simulink model "Airship_nonlinear_dynamics_simulink"  (R2024b)
settings: Solver=ode15s  StartTime=0.0  StopTime=1000  FixedStep=0.01  MaxStep=0.01  RelTol=1e-5  AbsTol=1e-8
InitFcn:
  | Init
values from neighbouring files (symbols this model uses):
  c = 0.465    [Init.m]    (also in Nonlinear_dynamics.m = 7; init_Skyship.m = 7)
  cf = 0.1395    [Init.m]    (also in Nonlinear_dynamics.m = 3; init_Skyship.m = 3)
  CL_alpha = 5.7    [Init.m]    (also in Nonlinear_dynamics.m; init_Skyship.m)
  D = 1.6    [Init.m]    (also in Nonlinear_dynamics.m = 14; init_Skyship.m = 14)
  delta = deg2rad(10)    [Nonlinear_dynamics.m]    (also in init_Skyship.m = -15)
  delta_e = 0    [Init.m]
  delta_r = 0    [Init.m]
  etaTDF = 1    [Init.m]    (also in Nonlinear_dynamics.m = 0.6; init_Skyship.m = 0.6)
  etaTP = 0.6    [Init.m]    (also in Nonlinear_dynamics.m; init_Skyship.m)
  fProp1 = 0    [Init.m]
  fProp2 = 0    [Init.m]
  fProp_max = 20    [Init.m]
  fTDF = 4000    [Nonlinear_dynamics.m]    (also in init_Skyship.m = 0)
  fTTP = 0    [Init.m]    (also in Nonlinear_dynamics.m = 2000; init_Skyship.m)
  FVN = [5, 5, 5]    [Init.m]    (also in Nonlinear_dynamics.m = 0; init_Skyship.m = 10)
  g = 9.81    [Init.m]    (also in Nonlinear_dynamics.m; init_Skyship.m)
  I33 = eye(3)    [Init.m]    (also in Nonlinear_dynamics.m; init_Skyship.m)
  Ixx = 1.7972    [Init.m]    (also in Nonlinear_dynamics.m = 200658; init_Skyship.m = 200658)
  Ixy = 0    [Init.m]    (also in Nonlinear_dynamics.m; init_Skyship.m)
  Ixz = 0    [Init.m]    (also in Nonlinear_dynamics.m; init_Skyship.m)
  Iyy = 4.9584    [Init.m]    (also in Nonlinear_dynamics.m = 850900; init_Skyship.m = 850900)
  Iyz = 0    [Init.m]    (also in Nonlinear_dynamics.m; init_Skyship.m)
  Izz = 7.9854    [Init.m]    (also in Nonlinear_dynamics.m = 649699; init_Skyship.m = 649699)
  k1 = keta(1)    [Init.m]    (also in Nonlinear_dynamics.m; init_Skyship.m = 0.08; ketaparameters.m = 0)
  k2 = keta(2)    [Init.m]    (also in Nonlinear_dynamics.m; init_Skyship.m = 0.89; ketaparameters.m = 0)
  k_dash = keta(3)    [Init.m]    (also in Nonlinear_dynamics.m; init_Skyship.m = 0.5; ketaparameters.m = 0)
  L = 4.7    [Init.m]    (also in Nonlinear_dynamics.m = zeros(1,4); init_Skyship.m = 52)
  m = 7.31    [Init.m]    (also in Nonlinear_dynamics.m = 5942; init_Skyship.m = 5942; velocity_tf_script.m; velocity_tf_script_v2.m)
  MAF = zeros(6,6)    [Init.m]    (also in Nonlinear_dynamics.m; init_Skyship.m)
  MVN = [0.2, 10, 5]    [Init.m]    (also in Nonlinear_dynamics.m = 0; init_Skyship.m = 0.001)
  p0 = 0    [Init.m]    (also in init_Skyship.m)
  phi0 = 0    [Init.m]    (also in init_Skyship.m)
  Prop1_alpha = 0    [Init.m]
  Prop2_alpha = 0    [Init.m]
  psi0 = 0    [Init.m]    (also in init_Skyship.m)
  q0 = 0    [Init.m]    (also in init_Skyship.m)
  r0 = 0    [Init.m]    (also in init_Skyship.m)
  rGxm = [XG-XB 0 ZG-ZB]'    [Init.m]    (also in Nonlinear_dynamics.m; init_Skyship.m)
  rho_0 = 1.225    [Init.m]    (also in Nonlinear_dynamics.m; init_Skyship.m)
  rho_he = 0.175    [Init.m]
  rTDF1 = [0 0.5 0]'    [Init.m]    (also in Nonlinear_dynamics.m = [3.5 7.87 21]'; init_Skyship.m = [3.5 7.87 21]')
  rTDF2 = [0 -0.5 0]'    [Init.m]    (also in Nonlinear_dynamics.m = [3.5 -7.87 21]'; init_Skyship.m = [3.5 -7.87 21]')
  rTTP = [0 0 0]'    [Init.m]    (also in Nonlinear_dynamics.m = [0 0 20.1]'; init_Skyship.m = [0 0 20.1]')
  Sf = 0.18135    [Init.m]    (also in Nonlinear_dynamics.m = 65; init_Skyship.m = 65)
  t_s = 0.005    [Init.m]
  theta0 = 1    [Init.m]    (also in init_Skyship.m = 0)
  u0 = 0.0    (= 0)    [Init.m]    (also in init_Skyship.m; velocity_tf_script.m = 4; velocity_tf_script_v2.m = 4)
  v0 = 0.0    (= 0)    [Init.m]    (also in init_Skyship.m)
  VB = 5.97    [Init.m]    (also in Nonlinear_dynamics.m = 5153; init_Skyship.m = 4911)
  w0 = 0.0    (= 0)    [Init.m]    (also in init_Skyship.m)
  xE0 = 0    [Init.m]    (also in init_Skyship.m)
  yE0 = 0    [Init.m]    (also in init_Skyship.m)
  zE0 = -h    (= -3.7495)    [Init.m]    (also in init_Skyship.m = -100)
undefined symbols (not defined in the file or in its folder): Sim3dSensor
libraries: slpidlib x13, simulink_extras x4, sim3dcameralib x1, sim3dlib x1, uavsim3dlib x1
(part 1 of 4)
settings Model: Creator=nicol  LastModifiedBy=nicol
settings DebuggingCC: ReadBeforeWriteMsg=DisableAll  WriteAfterWriteMsg=DisableAll  WriteAfterReadMsg=DisableAll  MultiTaskDSMMsg=none
settings ModelReferenceCC: UpdateModelReferenceTargets=IfOutOfDate
settings SFSimCC: SFSimEcho=off

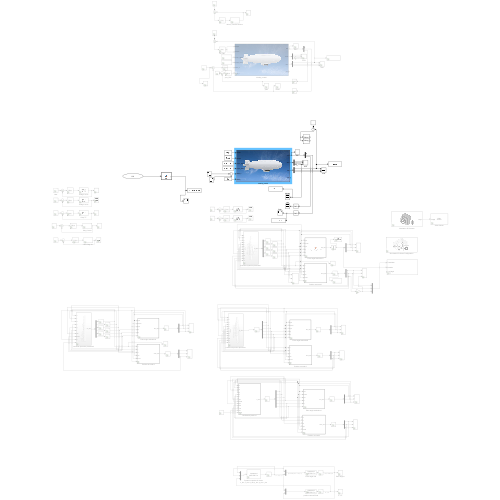
[thumbnail: Simulink's stored preview of the top-level diagram]
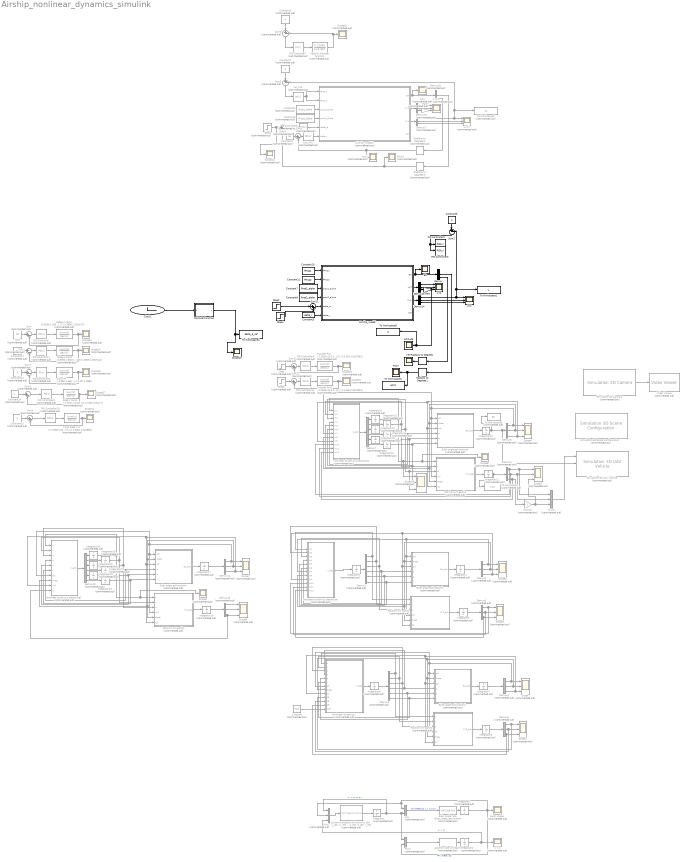
== system Airship_nonlinear_dynamics_simulink ==
  10deg 2 zeros : TransferFcn  Commented=on  Numerator=[0.8338 1.268]  Denominator=[1 0.3896 1.523e-07]
  10deg 3 zeros : TransferFcn  Commented=on  Numerator=[0.5955 1.938 0.5328]  Denominator=[1 0.9006 0.1659 0.0003742]
  "2 and 5deg mix " : TransferFcn  Commented=on  Numerator=[-0.1058 2.255]  Denominator=[1 0.6054 0.002888]
  5deg 2 zeros : TransferFcn  Commented=on  Numerator=[-0.3327 2.514]  Denominator=[1 0.7054 0.00177]
  Airship_model : Subsystem
      mask Display: image('istockphoto-184115621-612x612.jpg');
  Airship_model1 : Subsystem  Commented=on
      mask Display: image('istockphoto-184115621-612x612.jpg');
  Altitude : Scope
  Chirp TF : TransferFcn  Commented=on  Numerator=[-0.986 1.461]  Denominator=[1 1.237 0.3881]
  Clock1 : Clock
  Constant : Constant  Commented=on  Value=MAF
  Constant1 : Constant  Commented=on  Value=90
  Constant10 : Constant  Value=fProp1
  Constant11 : Constant  Value=fProp2
  Constant12 : Constant  Commented=on  Value=10
  Constant13 : Constant  Commented=on  Value=5
  Constant14 : Constant  Commented=on
  Constant15 : Constant  Commented=on
  Constant2 : Constant  Commented=on  Value=4
  Constant3 : Constant  Value=delta_r
  Constant4 : Constant  Commented=on  Value=Prop1_alpha
  Constant5 : Constant  Value=4
  Constant6 : Constant  Commented=on  Value=Prop2_alpha
  Constant7 : Constant  Value=Prop1_alpha
  Constant8 : Constant  Value=Prop2_alpha
  Constant9 : Constant  Commented=on  Value=4
  Demux : Demux  Outputs=3
  Demux{1,3,7,10} (4 alike) : Demux  Commented=on  Outputs=6
  Demux{2,4..6,8..9,11..12,15..17} (11 alike) : Demux  Commented=on  Outputs=3
  Demux13 : Demux  Outputs=3
  Demux14 : Demux  Outputs=3
  "Dynamic equation of motion u_dot, v_dot, w_dot, p_dot, q_dot, r_dot" : MATLABFcn  Commented=on  MATLABFcn=Nonlinear_dynamics  OutputDimensions=6
  EA : Scope
  EA1 : Scope  Commented=on
  Euler angle estimation1 : MATLAB Function  Commented=on  TreatAsAtomicUnit=on
  Euler angle estimation2 : MATLAB Function  Commented=on  TreatAsAtomicUnit=on
  Euler angle estimation3 : MATLAB Function  Commented=on  TreatAsAtomicUnit=on
  Euler angle estimation4 : MATLAB Function  Commented=on  TreatAsAtomicUnit=on
  Euler angle rate : MATLABFcn  Commented=on  MATLABFcn=Euler_angle_estimation  OutputDimensions=3
  Euler angles : Scope  Commented=on
  Gain : Gain  Gain=-1
  Gain2 : Gain  Commented=on  Gain=-1
  Integrator : Integrator  Commented=on  InitialCondition=[u0 v0 w0 p0 q0 r0]
  Integrator{1,4,7,10,17} (5 alike) : Integrator  Commented=on  InitialCondition=[phi0 theta0 psi0]
  Integrator{2,5,8,11,18} (5 alike) : Integrator  Commented=on  InitialCondition=[xE0 yE0 zE0]
  Integrator12 : Integrator  Commented=on  InitialCondition=v0
  Integrator13 : Integrator  Commented=on  InitialCondition=w0
  Integrator14 : Integrator  Commented=on  InitialCondition=p0
  Integrator15 : Integrator  Commented=on  InitialCondition=q0
  Integrator16 : Integrator  Commented=on  InitialCondition=r0
  Integrator19 : Integrator  Commented=on  InitialCondition=v0
  Integrator20 : Integrator  Commented=on  InitialCondition=w0
  Integrator21 : Integrator  Commented=on  InitialCondition=p0
  Integrator22 : Integrator  Commented=on  InitialCondition=q0
  Integrator23 : Integrator  Commented=on  InitialCondition=r0
  Integrator24 : Integrator  Commented=on  InitialCondition=u0
  Integrator3 : Integrator  Commented=on  InitialCondition=[u0 v0 w0 p0 q0 r0]
  Integrator6 : Integrator  Commented=on  InitialCondition=[u0 v0 w0 p0 q0 r0]
  Integrator9 : Integrator  Commented=on  InitialCondition=u0
  MATLAB Function : MATLAB Function  TreatAsAtomicUnit=on  SystemSampleTime=0.001
  Multiply : Gain  Commented=on  Gain=-1
  Mux : Mux  Commented=on  Inputs=2
  Mux1 : Mux  Commented=on  Inputs=2
  Mux2 : Mux  Commented=on  Inputs=3
  Mux3 : Mux  Commented=on  Inputs=3
  Nonlinear dynamics1 : MATLAB Function  Commented=on  TreatAsAtomicUnit=on
  PID Controller : slpidlib/PID Controller  Commented=on  Controller=PD  Form=Parallel  TimeDomain=Continuous-time  UseExternalTs=off  SampleTime=-1  IntegratorMethod=Forward Euler  FilterMethod=Forward Euler  ControllerParametersSource=internal  P=8.41897155293235  I=0.0815373305653461  UseKiTs=off  D=0.61435415222299  UseExternalDerivativeSource=off  N=10.82924204586  UseFilter=on  TunerSelectOption=Transfer Function Based (PID Tuner App)  InitialConditionSource=internal  InitialConditionForIntegrator=0  InitialConditionForFilter=0  DifferentiatorICPrevScaledInput=0  ExternalReset=none  TrackingMode=off  Kt=1  LimitOutput=off  SatLimitsSource=internal  UpperSaturationLimit=inf  LowerSaturationLimit=-inf  LinearizeAsGain=on  AntiWindupMode=none  Kb=1  LimitIntegrator=off  UpperIntegratorSaturationLimit=inf  LowerIntegratorSaturationLimit=-inf  POutMin=[]  POutMax=[]  IOutMin=[]  IOutMax=[]  DOutMin=[]  DOutMax=[]  NOutMin=[]  NOutMax=[]  SumOutMin=[]  SumOutMax=[]  SaturationOutMin=[]  SaturationOutMax=[]  PParamMin=[]  PParamMax=[]  IParamMin=[]  IParamMax=[]  DParamMin=[]  DParamMax=[]  NParamMin=[]  NParamMax=[]  KbParamMin=[]  KbParamMax=[]  KtParamMin=[]  KtParamMax=[]  KbOutMin=[]  KbOutMax=[]  KtOutMin=[]  KtOutMax=[]  IntegratorOutMin=[]  IntegratorOutMax=[]  FilterOutMin=[]  FilterOutMax=[]  SumI1OutMin=[]  SumI1OutMax=[]  SumI2OutMin=[]  SumI2OutMax=[]  SumI3OutMin=[]  SumI3OutMax=[]  SumI4OutMin=[]  SumI4OutMax=[]  SumDOutMin=[]  SumDOutMax=[]  DifferentiatorOutMin=[]  DifferentiatorOutMax=[]  FilterDiffOutCoefMin=[]  FilterDiffOutCoefMax=[]  ReciprocalOutMin=[]  ReciprocalOutMax=[]  SumDenOutMin=[]  SumDenOutMax=[]  SumNumOutMin=[]  SumNumOutMax=[]  DivideOutMin=[]  DivideOutMax=[]  UdiffTsProdOutMin=[]  UdiffTsProdOutMax=[]  NTsProdOutMin=[]  NTsProdOutMax=[]  UintegralTsProdOutMin=[]  UintegralTsProdOutMax=[]  UngainTsProdOutMin=[]  UngainTsProdOutMax=[]  ClampingZeroOutDataTypeStr=Inherit: Inherit via back propagation  ClampingZeroOutMin=[]  ClampingZeroOutMax=[]  FilterDenConstantOutDataTypeStr=Inherit: Inherit via back propagation  FilterDenConstantOutMin=[]  FilterDenConstantOutMax=[]  PCopyOutDataTypeStr=Inherit: Inherit via back propagation  PCopyOutMin=[]  PCopyOutMax=[]  NCopyOutDataTypeStr=Inherit: Inherit via back propagation  NCopyOutMin=[]  NCopyOutMax=[]  IntegratorContinuousStateAttributes=''  IntegratorStateMustResolveToSignalObject=off  IntegratorRTWStateStorageClass=Auto  FilterContinuousStateAttributes=''  FilterStateMustResolveToSignalObject=off  FilterRTWStateStorageClass=Auto  ParallelPVariant=InternalParameters  IdealPVariant=Disabled  IVariant=Disabled  DVariant=InternalParameters  IntegratorVariant=Disabled  SatVariant=Disabled  AWVariant=Disabled  PCopyVariant=Disabled  TRVariant=Disabled  FdbkBlocksVariant=Forward  IdealPFdbkVariant=Disabled  SatFdbkVariant=Disabled  DerivativeFilterVariant=ContFilter  NVariant=InternalParameters  NCopyVariant=Disabled  FilterICVariant=InternalICsFilter  IntegratorICVariant=Disabled  ExternalResetVariant=Disabled  TRSumVariant=Passthrough  SumFdbkVariant=Disabled  SumVariant=Sum_PD  TsampFilterVariant=InternalTs  TsampNgainVariant=Passthrough  TsampIntegralVariant=Disabled_SignalSpec  ExternalSaturationOutDataTypeStr=Inherit: Same as second input  DerivativeSourceVariant=ErrorSignal  PreIntVariant=InternalPreInt
  PID Controller1 : slpidlib/PID Controller  Commented=on  Controller=PD  Form=Parallel  TimeDomain=Continuous-time  UseExternalTs=off  SampleTime=-1  IntegratorMethod=Forward Euler  FilterMethod=Forward Euler  ControllerParametersSource=internal  P=26.8682  I=0.0815373305653461  UseKiTs=off  D=7.9856  UseExternalDerivativeSource=off  N=4.34708219903778  UseFilter=on  TunerSelectOption=Transfer Function Based (PID Tuner App)  InitialConditionSource=internal  InitialConditionForIntegrator=0  InitialConditionForFilter=0  DifferentiatorICPrevScaledInput=0  ExternalReset=none  TrackingMode=off  Kt=1  LimitOutput=off  SatLimitsSource=internal  UpperSaturationLimit=inf  LowerSaturationLimit=-inf  LinearizeAsGain=on  AntiWindupMode=none  Kb=1  LimitIntegrator=off  UpperIntegratorSaturationLimit=inf  LowerIntegratorSaturationLimit=-inf  POutMin=[]  POutMax=[]  IOutMin=[]  IOutMax=[]  DOutMin=[]  DOutMax=[]  NOutMin=[]  NOutMax=[]  SumOutMin=[]  SumOutMax=[]  SaturationOutMin=[]  SaturationOutMax=[]  PParamMin=[]  PParamMax=[]  IParamMin=[]  IParamMax=[]  DParamMin=[]  DParamMax=[]  NParamMin=[]  NParamMax=[]  KbParamMin=[]  KbParamMax=[]  KtParamMin=[]  KtParamMax=[]  KbOutMin=[]  KbOutMax=[]  KtOutMin=[]  KtOutMax=[]  IntegratorOutMin=[]  IntegratorOutMax=[]  FilterOutMin=[]  FilterOutMax=[]  SumI1OutMin=[]  SumI1OutMax=[]  SumI2OutMin=[]  SumI2OutMax=[]  SumI3OutMin=[]  SumI3OutMax=[]  SumI4OutMin=[]  SumI4OutMax=[]  SumDOutMin=[]  SumDOutMax=[]  DifferentiatorOutMin=[]  DifferentiatorOutMax=[]  FilterDiffOutCoefMin=[]  FilterDiffOutCoefMax=[]  ReciprocalOutMin=[]  ReciprocalOutMax=[]  SumDenOutMin=[]  SumDenOutMax=[]  SumNumOutMin=[]  SumNumOutMax=[]  DivideOutMin=[]  DivideOutMax=[]  UdiffTsProdOutMin=[]  UdiffTsProdOutMax=[]  NTsProdOutMin=[]  NTsProdOutMax=[]  UintegralTsProdOutMin=[]  UintegralTsProdOutMax=[]  UngainTsProdOutMin=[]  UngainTsProdOutMax=[]  ClampingZeroOutDataTypeStr=Inherit: Inherit via back propagation  ClampingZeroOutMin=[]  ClampingZeroOutMax=[]  FilterDenConstantOutDataTypeStr=Inherit: Inherit via back propagation  FilterDenConstantOutMin=[]  FilterDenConstantOutMax=[]  PCopyOutDataTypeStr=Inherit: Inherit via back propagation  PCopyOutMin=[]  PCopyOutMax=[]  NCopyOutDataTypeStr=Inherit: Inherit via back propagation  NCopyOutMin=[]  NCopyOutMax=[]  IntegratorContinuousStateAttributes=''  IntegratorStateMustResolveToSignalObject=off  IntegratorRTWStateStorageClass=Auto  FilterContinuousStateAttributes=''  FilterStateMustResolveToSignalObject=off  FilterRTWStateStorageClass=Auto  ParallelPVariant=InternalParameters  IdealPVariant=Disabled  IVariant=Disabled  DVariant=InternalParameters  IntegratorVariant=Disabled  SatVariant=Disabled  AWVariant=Disabled  PCopyVariant=Disabled  TRVariant=Disabled  FdbkBlocksVariant=Forward  IdealPFdbkVariant=Disabled  SatFdbkVariant=Disabled  DerivativeFilterVariant=ContFilter  NVariant=InternalParameters  NCopyVariant=Disabled  FilterICVariant=InternalICsFilter  IntegratorICVariant=Disabled  ExternalResetVariant=Disabled  TRSumVariant=Passthrough  SumFdbkVariant=Disabled  SumVariant=Sum_PD  TsampFilterVariant=InternalTs  TsampNgainVariant=Passthrough  TsampIntegralVariant=Disabled_SignalSpec  ExternalSaturationOutDataTypeStr=Inherit: Same as second input  DerivativeSourceVariant=ErrorSignal  PreIntVariant=InternalPreInt
  PID Controller10 : slpidlib/PID Controller  Commented=on  Controller=PID  Form=Parallel  TimeDomain=Continuous-time  UseExternalTs=off  SampleTime=-1  IntegratorMethod=Forward Euler  FilterMethod=Forward Euler  ControllerParametersSource=internal  P=0.115369751085597  I=0.002  UseKiTs=off  D=0.178743752919418  UseExternalDerivativeSource=off  N=1.68043173640321  UseFilter=on  TunerSelectOption=Transfer Function Based (PID Tuner App)  InitialConditionSource=internal  InitialConditionForIntegrator=0  InitialConditionForFilter=0  DifferentiatorICPrevScaledInput=0  ExternalReset=none  TrackingMode=off  Kt=1  LimitOutput=off  SatLimitsSource=internal  UpperSaturationLimit=inf  LowerSaturationLimit=-inf  LinearizeAsGain=on  AntiWindupMode=none  Kb=1  LimitIntegrator=off  UpperIntegratorSaturationLimit=inf  LowerIntegratorSaturationLimit=-inf  POutMin=[]  POutMax=[]  IOutMin=[]  IOutMax=[]  DOutMin=[]  DOutMax=[]  NOutMin=[]  NOutMax=[]  SumOutMin=[]  SumOutMax=[]  SaturationOutMin=[]  SaturationOutMax=[]  PParamMin=[]  PParamMax=[]  IParamMin=[]  IParamMax=[]  DParamMin=[]  DParamMax=[]  NParamMin=[]  NParamMax=[]  KbParamMin=[]  KbParamMax=[]  KtParamMin=[]  KtParamMax=[]  KbOutMin=[]  KbOutMax=[]  KtOutMin=[]  KtOutMax=[]  IntegratorOutMin=[]  IntegratorOutMax=[]  FilterOutMin=[]  FilterOutMax=[]  SumI1OutMin=[]  SumI1OutMax=[]  SumI2OutMin=[]  SumI2OutMax=[]  SumI3OutMin=[]  SumI3OutMax=[]  SumI4OutMin=[]  SumI4OutMax=[]  SumDOutMin=[]  SumDOutMax=[]  DifferentiatorOutMin=[]  DifferentiatorOutMax=[]  FilterDiffOutCoefMin=[]  FilterDiffOutCoefMax=[]  ReciprocalOutMin=[]  ReciprocalOutMax=[]  SumDenOutMin=[]  SumDenOutMax=[]  SumNumOutMin=[]  SumNumOutMax=[]  DivideOutMin=[]  DivideOutMax=[]  UdiffTsProdOutMin=[]  UdiffTsProdOutMax=[]  NTsProdOutMin=[]  NTsProdOutMax=[]  UintegralTsProdOutMin=[]  UintegralTsProdOutMax=[]  UngainTsProdOutMin=[]  UngainTsProdOutMax=[]  ClampingZeroOutDataTypeStr=Inherit: Inherit via back propagation  ClampingZeroOutMin=[]  ClampingZeroOutMax=[]  FilterDenConstantOutDataTypeStr=Inherit: Inherit via back propagation  FilterDenConstantOutMin=[]  FilterDenConstantOutMax=[]  PCopyOutDataTypeStr=Inherit: Inherit via back propagation  PCopyOutMin=[]  PCopyOutMax=[]  NCopyOutDataTypeStr=Inherit: Inherit via back propagation  NCopyOutMin=[]  NCopyOutMax=[]  IntegratorContinuousStateAttributes=''  IntegratorStateMustResolveToSignalObject=off  IntegratorRTWStateStorageClass=Auto  FilterContinuousStateAttributes=''  FilterStateMustResolveToSignalObject=off  FilterRTWStateStorageClass=Auto  ParallelPVariant=InternalParameters  IdealPVariant=Disabled  IVariant=InternalParameters  DVariant=InternalParameters  IntegratorVariant=Continuous  SatVariant=Disabled  AWVariant=Passthrough  PCopyVariant=Disabled  TRVariant=Disabled  FdbkBlocksVariant=Forward  IdealPFdbkVariant=Disabled  SatFdbkVariant=Disabled  DerivativeFilterVariant=ContFilter  NVariant=InternalParameters  NCopyVariant=Disabled  FilterICVariant=InternalICsFilter  IntegratorICVariant=InternalICs  ExternalResetVariant=Disabled  TRSumVariant=Passthrough  SumFdbkVariant=Disabled  SumVariant=Sum_PID  TsampFilterVariant=InternalTs  TsampNgainVariant=Passthrough  TsampIntegralVariant=Disabled_SignalSpec  ExternalSaturationOutDataTypeStr=Inherit: Same as second input  DerivativeSourceVariant=ErrorSignal  PreIntVariant=InternalPreInt
  PID Controller11 : slpidlib/PID Controller  Commented=on  Controller=PD  Form=Parallel  TimeDomain=Continuous-time  UseExternalTs=off  SampleTime=-1  IntegratorMethod=Forward Euler  FilterMethod=Forward Euler  ControllerParametersSource=internal  P=-1948.3682  I=1  UseKiTs=off  D=3565.5139  UseExternalDerivativeSource=off  N=100  UseFilter=on  TunerSelectOption=Transfer Function Based (PID Tuner App)  InitialConditionSource=internal  InitialConditionForIntegrator=0  InitialConditionForFilter=0  DifferentiatorICPrevScaledInput=0  ExternalReset=none  TrackingMode=off  Kt=1  LimitOutput=off  SatLimitsSource=internal  UpperSaturationLimit=inf  LowerSaturationLimit=-inf  LinearizeAsGain=on  AntiWindupMode=none  Kb=1  LimitIntegrator=off  UpperIntegratorSaturationLimit=inf  LowerIntegratorSaturationLimit=-inf  POutMin=[]  POutMax=[]  IOutMin=[]  IOutMax=[]  DOutMin=[]  DOutMax=[]  NOutMin=[]  NOutMax=[]  SumOutMin=[]  SumOutMax=[]  SaturationOutMin=[]  SaturationOutMax=[]  PParamMin=[]  PParamMax=[]  IParamMin=[]  IParamMax=[]  DParamMin=[]  DParamMax=[]  NParamMin=[]  NParamMax=[]  KbParamMin=[]  KbParamMax=[]  KtParamMin=[]  KtParamMax=[]  KbOutMin=[]  KbOutMax=[]  KtOutMin=[]  KtOutMax=[]  IntegratorOutMin=[]  IntegratorOutMax=[]  FilterOutMin=[]  FilterOutMax=[]  SumI1OutMin=[]  SumI1OutMax=[]  SumI2OutMin=[]  SumI2OutMax=[]  SumI3OutMin=[]  SumI3OutMax=[]  SumI4OutMin=[]  SumI4OutMax=[]  SumDOutMin=[]  SumDOutMax=[]  DifferentiatorOutMin=[]  DifferentiatorOutMax=[]  FilterDiffOutCoefMin=[]  FilterDiffOutCoefMax=[]  ReciprocalOutMin=[]  ReciprocalOutMax=[]  SumDenOutMin=[]  SumDenOutMax=[]  SumNumOutMin=[]  SumNumOutMax=[]  DivideOutMin=[]  DivideOutMax=[]  UdiffTsProdOutMin=[]  UdiffTsProdOutMax=[]  NTsProdOutMin=[]  NTsProdOutMax=[]  UintegralTsProdOutMin=[]  UintegralTsProdOutMax=[]  UngainTsProdOutMin=[]  UngainTsProdOutMax=[]  ClampingZeroOutDataTypeStr=Inherit: Inherit via back propagation  ClampingZeroOutMin=[]  ClampingZeroOutMax=[]  FilterDenConstantOutDataTypeStr=Inherit: Inherit via back propagation  FilterDenConstantOutMin=[]  FilterDenConstantOutMax=[]  PCopyOutDataTypeStr=Inherit: Inherit via back propagation  PCopyOutMin=[]  PCopyOutMax=[]  NCopyOutDataTypeStr=Inherit: Inherit via back propagation  NCopyOutMin=[]  NCopyOutMax=[]  IntegratorContinuousStateAttributes=''  IntegratorStateMustResolveToSignalObject=off  IntegratorRTWStateStorageClass=Auto  FilterContinuousStateAttributes=''  FilterStateMustResolveToSignalObject=off  FilterRTWStateStorageClass=Auto  ParallelPVariant=InternalParameters  IdealPVariant=Disabled  IVariant=Disabled  DVariant=InternalParameters  IntegratorVariant=Disabled  SatVariant=Disabled  AWVariant=Disabled  PCopyVariant=Disabled  TRVariant=Disabled  FdbkBlocksVariant=Forward  IdealPFdbkVariant=Disabled  SatFdbkVariant=Disabled  DerivativeFilterVariant=ContFilter  NVariant=InternalParameters  NCopyVariant=Disabled  FilterICVariant=InternalICsFilter  IntegratorICVariant=Disabled  ExternalResetVariant=Disabled  TRSumVariant=Passthrough  SumFdbkVariant=Disabled  SumVariant=Sum_PD  TsampFilterVariant=InternalTs  TsampNgainVariant=Passthrough  TsampIntegralVariant=Disabled_SignalSpec  ExternalSaturationOutDataTypeStr=Inherit: Same as second input  DerivativeSourceVariant=ErrorSignal  PreIntVariant=InternalPreInt
  PID Controller2 : slpidlib/PID Controller  Controller=PID  Form=Parallel  TimeDomain=Continuous-time  UseExternalTs=off  SampleTime=-1  IntegratorMethod=Forward Euler  FilterMethod=Forward Euler  ControllerParametersSource=internal  P=38.251  I=3.3468  UseKiTs=off  D=0.033416  UseExternalDerivativeSource=off  N=1142.828  UseFilter=on  TunerSelectOption=Transfer Function Based (PID Tuner App)  InitialConditionSource=internal  InitialConditionForIntegrator=0  InitialConditionForFilter=0  DifferentiatorICPrevScaledInput=0  ExternalReset=none  TrackingMode=off  Kt=1  LimitOutput=off  SatLimitsSource=internal  UpperSaturationLimit=inf  LowerSaturationLimit=-inf  LinearizeAsGain=on  AntiWindupMode=none  Kb=1  LimitIntegrator=off  UpperIntegratorSaturationLimit=inf  LowerIntegratorSaturationLimit=-inf  POutMin=[]  POutMax=[]  IOutMin=[]  IOutMax=[]  DOutMin=[]  DOutMax=[]  NOutMin=[]  NOutMax=[]  SumOutMin=[]  SumOutMax=[]  SaturationOutMin=[]  SaturationOutMax=[]  PParamMin=[]  PParamMax=[]  IParamMin=[]  IParamMax=[]  DParamMin=[]  DParamMax=[]  NParamMin=[]  NParamMax=[]  KbParamMin=[]  KbParamMax=[]  KtParamMin=[]  KtParamMax=[]  KbOutMin=[]  KbOutMax=[]  KtOutMin=[]  KtOutMax=[]  IntegratorOutMin=[]  IntegratorOutMax=[]  FilterOutMin=[]  FilterOutMax=[]  SumI1OutMin=[]  SumI1OutMax=[]  SumI2OutMin=[]  SumI2OutMax=[]  SumI3OutMin=[]  SumI3OutMax=[]  SumI4OutMin=[]  SumI4OutMax=[]  SumDOutMin=[]  SumDOutMax=[]  DifferentiatorOutMin=[]  DifferentiatorOutMax=[]  FilterDiffOutCoefMin=[]  FilterDiffOutCoefMax=[]  ReciprocalOutMin=[]  ReciprocalOutMax=[]  SumDenOutMin=[]  SumDenOutMax=[]  SumNumOutMin=[]  SumNumOutMax=[]  DivideOutMin=[]  DivideOutMax=[]  UdiffTsProdOutMin=[]  UdiffTsProdOutMax=[]  NTsProdOutMin=[]  NTsProdOutMax=[]  UintegralTsProdOutMin=[]  UintegralTsProdOutMax=[]  UngainTsProdOutMin=[]  UngainTsProdOutMax=[]  ClampingZeroOutDataTypeStr=Inherit: Inherit via back propagation  ClampingZeroOutMin=[]  ClampingZeroOutMax=[]  FilterDenConstantOutDataTypeStr=Inherit: Inherit via back propagation  FilterDenConstantOutMin=[]  FilterDenConstantOutMax=[]  PCopyOutDataTypeStr=Inherit: Inherit via back propagation  PCopyOutMin=[]  PCopyOutMax=[]  NCopyOutDataTypeStr=Inherit: Inherit via back propagation  NCopyOutMin=[]  NCopyOutMax=[]  IntegratorContinuousStateAttributes=''  IntegratorStateMustResolveToSignalObject=off  IntegratorRTWStateStorageClass=Auto  FilterContinuousStateAttributes=''  FilterStateMustResolveToSignalObject=off  FilterRTWStateStorageClass=Auto  ParallelPVariant=InternalParameters  IdealPVariant=Disabled  IVariant=InternalParameters  DVariant=InternalParameters  IntegratorVariant=Continuous  SatVariant=Disabled  AWVariant=Passthrough  PCopyVariant=Disabled  TRVariant=Disabled  FdbkBlocksVariant=Forward  IdealPFdbkVariant=Disabled  SatFdbkVariant=Disabled  DerivativeFilterVariant=ContFilter  NVariant=InternalParameters  NCopyVariant=Disabled  FilterICVariant=InternalICsFilter  IntegratorICVariant=InternalICs  ExternalResetVariant=Disabled  TRSumVariant=Passthrough  SumFdbkVariant=Disabled  SumVariant=Sum_PID  TsampFilterVariant=InternalTs  TsampNgainVariant=Passthrough  TsampIntegralVariant=Disabled_SignalSpec  ExternalSaturationOutDataTypeStr=Inherit: Same as second input  DerivativeSourceVariant=ErrorSignal  PreIntVariant=InternalPreInt
  PID Controller3 : slpidlib/PID Controller  Controller=PID  Form=Parallel  TimeDomain=Continuous-time  UseExternalTs=off  SampleTime=-1  IntegratorMethod=Forward Euler  FilterMethod=Forward Euler  ControllerParametersSource=internal  P=38.251  I=3.3468  UseKiTs=off  D=0.033416  UseExternalDerivativeSource=off  N=1142.828  UseFilter=on  TunerSelectOption=Transfer Function Based (PID Tuner App)  InitialConditionSource=internal  InitialConditionForIntegrator=0  InitialConditionForFilter=0  DifferentiatorICPrevScaledInput=0  ExternalReset=none  TrackingMode=off  Kt=1  LimitOutput=off  SatLimitsSource=internal  UpperSaturationLimit=inf  LowerSaturationLimit=-inf  LinearizeAsGain=on  AntiWindupMode=none  Kb=1  LimitIntegrator=off  UpperIntegratorSaturationLimit=inf  LowerIntegratorSaturationLimit=-inf  POutMin=[]  POutMax=[]  IOutMin=[]  IOutMax=[]  DOutMin=[]  DOutMax=[]  NOutMin=[]  NOutMax=[]  SumOutMin=[]  SumOutMax=[]  SaturationOutMin=[]  SaturationOutMax=[]  PParamMin=[]  PParamMax=[]  IParamMin=[]  IParamMax=[]  DParamMin=[]  DParamMax=[]  NParamMin=[]  NParamMax=[]  KbParamMin=[]  KbParamMax=[]  KtParamMin=[]  KtParamMax=[]  KbOutMin=[]  KbOutMax=[]  KtOutMin=[]  KtOutMax=[]  IntegratorOutMin=[]  IntegratorOutMax=[]  FilterOutMin=[]  FilterOutMax=[]  SumI1OutMin=[]  SumI1OutMax=[]  SumI2OutMin=[]  SumI2OutMax=[]  SumI3OutMin=[]  SumI3OutMax=[]  SumI4OutMin=[]  SumI4OutMax=[]  SumDOutMin=[]  SumDOutMax=[]  DifferentiatorOutMin=[]  DifferentiatorOutMax=[]  FilterDiffOutCoefMin=[]  FilterDiffOutCoefMax=[]  ReciprocalOutMin=[]  ReciprocalOutMax=[]  SumDenOutMin=[]  SumDenOutMax=[]  SumNumOutMin=[]  SumNumOutMax=[]  DivideOutMin=[]  DivideOutMax=[]  UdiffTsProdOutMin=[]  UdiffTsProdOutMax=[]  NTsProdOutMin=[]  NTsProdOutMax=[]  UintegralTsProdOutMin=[]  UintegralTsProdOutMax=[]  UngainTsProdOutMin=[]  UngainTsProdOutMax=[]  ClampingZeroOutDataTypeStr=Inherit: Inherit via back propagation  ClampingZeroOutMin=[]  ClampingZeroOutMax=[]  FilterDenConstantOutDataTypeStr=Inherit: Inherit via back propagation  FilterDenConstantOutMin=[]  FilterDenConstantOutMax=[]  PCopyOutDataTypeStr=Inherit: Inherit via back propagation  PCopyOutMin=[]  PCopyOutMax=[]  NCopyOutDataTypeStr=Inherit: Inherit via back propagation  NCopyOutMin=[]  NCopyOutMax=[]  IntegratorContinuousStateAttributes=''  IntegratorStateMustResolveToSignalObject=off  IntegratorRTWStateStorageClass=Auto  FilterContinuousStateAttributes=''  FilterStateMustResolveToSignalObject=off  FilterRTWStateStorageClass=Auto  ParallelPVariant=InternalParameters  IdealPVariant=Disabled  IVariant=InternalParameters  DVariant=InternalParameters  IntegratorVariant=Continuous  SatVariant=Disabled  AWVariant=Passthrough  PCopyVariant=Disabled  TRVariant=Disabled  FdbkBlocksVariant=Forward  IdealPFdbkVariant=Disabled  SatFdbkVariant=Disabled  DerivativeFilterVariant=ContFilter  NVariant=InternalParameters  NCopyVariant=Disabled  FilterICVariant=InternalICsFilter  IntegratorICVariant=InternalICs  ExternalResetVariant=Disabled  TRSumVariant=Passthrough  SumFdbkVariant=Disabled  SumVariant=Sum_PID  TsampFilterVariant=InternalTs  TsampNgainVariant=Passthrough  TsampIntegralVariant=Disabled_SignalSpec  ExternalSaturationOutDataTypeStr=Inherit: Same as second input  DerivativeSourceVariant=ErrorSignal  PreIntVariant=InternalPreInt
  PID Controller4 : slpidlib/PID Controller  Commented=on  Controller=PD  Form=Parallel  TimeDomain=Continuous-time  UseExternalTs=off  SampleTime=-1  IntegratorMethod=Forward Euler  FilterMethod=Forward Euler  ControllerParametersSource=internal  P=36.845690528866  I=1  UseKiTs=off  D=109.426646231735  UseExternalDerivativeSource=off  N=199.408721868741  UseFilter=on  TunerSelectOption=Transfer Function Based (PID Tuner App)  InitialConditionSource=internal  InitialConditionForIntegrator=0  InitialConditionForFilter=0  DifferentiatorICPrevScaledInput=0  ExternalReset=none  TrackingMode=off  Kt=1  LimitOutput=off  SatLimitsSource=internal  UpperSaturationLimit=inf  LowerSaturationLimit=-inf  LinearizeAsGain=on  AntiWindupMode=none  Kb=1  LimitIntegrator=off  UpperIntegratorSaturationLimit=inf  LowerIntegratorSaturationLimit=-inf  POutMin=[]  POutMax=[]  IOutMin=[]  IOutMax=[]  DOutMin=[]  DOutMax=[]  NOutMin=[]  NOutMax=[]  SumOutMin=[]  SumOutMax=[]  SaturationOutMin=[]  SaturationOutMax=[]  PParamMin=[]  PParamMax=[]  IParamMin=[]  IParamMax=[]  DParamMin=[]  DParamMax=[]  NParamMin=[]  NParamMax=[]  KbParamMin=[]  KbParamMax=[]  KtParamMin=[]  KtParamMax=[]  KbOutMin=[]  KbOutMax=[]  KtOutMin=[]  KtOutMax=[]  IntegratorOutMin=[]  IntegratorOutMax=[]  FilterOutMin=[]  FilterOutMax=[]  SumI1OutMin=[]  SumI1OutMax=[]  SumI2OutMin=[]  SumI2OutMax=[]  SumI3OutMin=[]  SumI3OutMax=[]  SumI4OutMin=[]  SumI4OutMax=[]  SumDOutMin=[]  SumDOutMax=[]  DifferentiatorOutMin=[]  DifferentiatorOutMax=[]  FilterDiffOutCoefMin=[]  FilterDiffOutCoefMax=[]  ReciprocalOutMin=[]  ReciprocalOutMax=[]  SumDenOutMin=[]  SumDenOutMax=[]  SumNumOutMin=[]  SumNumOutMax=[]  DivideOutMin=[]  DivideOutMax=[]  UdiffTsProdOutMin=[]  UdiffTsProdOutMax=[]  NTsProdOutMin=[]  NTsProdOutMax=[]  UintegralTsProdOutMin=[]  UintegralTsProdOutMax=[]  UngainTsProdOutMin=[]  UngainTsProdOutMax=[]  ClampingZeroOutDataTypeStr=Inherit: Inherit via back propagation  ClampingZeroOutMin=[]  ClampingZeroOutMax=[]  FilterDenConstantOutDataTypeStr=Inherit: Inherit via back propagation  FilterDenConstantOutMin=[]  FilterDenConstantOutMax=[]  PCopyOutDataTypeStr=Inherit: Inherit via back propagation  PCopyOutMin=[]  PCopyOutMax=[]  NCopyOutDataTypeStr=Inherit: Inherit via back propagation  NCopyOutMin=[]  NCopyOutMax=[]  IntegratorContinuousStateAttributes=''  IntegratorStateMustResolveToSignalObject=off  IntegratorRTWStateStorageClass=Auto  FilterContinuousStateAttributes=''  FilterStateMustResolveToSignalObject=off  FilterRTWStateStorageClass=Auto  ParallelPVariant=InternalParameters  IdealPVariant=Disabled  IVariant=Disabled  DVariant=InternalParameters  IntegratorVariant=Disabled  SatVariant=Disabled  AWVariant=Disabled  PCopyVariant=Disabled  TRVariant=Disabled  FdbkBlocksVariant=Forward  IdealPFdbkVariant=Disabled  SatFdbkVariant=Disabled  DerivativeFilterVariant=ContFilter  NVariant=InternalParameters  NCopyVariant=Disabled  FilterICVariant=InternalICsFilter  IntegratorICVariant=Disabled  ExternalResetVariant=Disabled  TRSumVariant=Passthrough  SumFdbkVariant=Disabled  SumVariant=Sum_PD  TsampFilterVariant=InternalTs  TsampNgainVariant=Passthrough  TsampIntegralVariant=Disabled_SignalSpec  ExternalSaturationOutDataTypeStr=Inherit: Same as second input  DerivativeSourceVariant=ErrorSignal  PreIntVariant=InternalPreInt
  PID Controller5 : slpidlib/PID Controller  Commented=on  Controller=PID  Form=Parallel  TimeDomain=Continuous-time  UseExternalTs=off  SampleTime=-1  IntegratorMethod=Forward Euler  FilterMethod=Forward Euler  ControllerParametersSource=internal  P=10  I=0  UseKiTs=off  D=0  UseExternalDerivativeSource=off  N=100  UseFilter=on  TunerSelectOption=Transfer Function Based (PID Tuner App)  InitialConditionSource=internal  InitialConditionForIntegrator=0  InitialConditionForFilter=0  DifferentiatorICPrevScaledInput=0  ExternalReset=none  TrackingMode=off  Kt=1  LimitOutput=off  SatLimitsSource=internal  UpperSaturationLimit=inf  LowerSaturationLimit=-inf  LinearizeAsGain=on  AntiWindupMode=none  Kb=1  LimitIntegrator=off  UpperIntegratorSaturationLimit=inf  LowerIntegratorSaturationLimit=-inf  POutMin=[]  POutMax=[]  IOutMin=[]  IOutMax=[]  DOutMin=[]  DOutMax=[]  NOutMin=[]  NOutMax=[]  SumOutMin=[]  SumOutMax=[]  SaturationOutMin=[]  SaturationOutMax=[]  PParamMin=[]  PParamMax=[]  IParamMin=[]  IParamMax=[]  DParamMin=[]  DParamMax=[]  NParamMin=[]  NParamMax=[]  KbParamMin=[]  KbParamMax=[]  KtParamMin=[]  KtParamMax=[]  KbOutMin=[]  KbOutMax=[]  KtOutMin=[]  KtOutMax=[]  IntegratorOutMin=[]  IntegratorOutMax=[]  FilterOutMin=[]  FilterOutMax=[]  SumI1OutMin=[]  SumI1OutMax=[]  SumI2OutMin=[]  SumI2OutMax=[]  SumI3OutMin=[]  SumI3OutMax=[]  SumI4OutMin=[]  SumI4OutMax=[]  SumDOutMin=[]  SumDOutMax=[]  DifferentiatorOutMin=[]  DifferentiatorOutMax=[]  FilterDiffOutCoefMin=[]  FilterDiffOutCoefMax=[]  ReciprocalOutMin=[]  ReciprocalOutMax=[]  SumDenOutMin=[]  SumDenOutMax=[]  SumNumOutMin=[]  SumNumOutMax=[]  DivideOutMin=[]  DivideOutMax=[]  UdiffTsProdOutMin=[]  UdiffTsProdOutMax=[]  NTsProdOutMin=[]  NTsProdOutMax=[]  UintegralTsProdOutMin=[]  UintegralTsProdOutMax=[]  UngainTsProdOutMin=[]  UngainTsProdOutMax=[]  ClampingZeroOutDataTypeStr=Inherit: Inherit via back propagation  ClampingZeroOutMin=[]  ClampingZeroOutMax=[]  FilterDenConstantOutDataTypeStr=Inherit: Inherit via back propagation  FilterDenConstantOutMin=[]  FilterDenConstantOutMax=[]  PCopyOutDataTypeStr=Inherit: Inherit via back propagation  PCopyOutMin=[]  PCopyOutMax=[]  NCopyOutDataTypeStr=Inherit: Inherit via back propagation  NCopyOutMin=[]  NCopyOutMax=[]  IntegratorContinuousStateAttributes=''  IntegratorStateMustResolveToSignalObject=off  IntegratorRTWStateStorageClass=Auto  FilterContinuousStateAttributes=''  FilterStateMustResolveToSignalObject=off  FilterRTWStateStorageClass=Auto  ParallelPVariant=InternalParameters  IdealPVariant=Disabled  IVariant=InternalParameters  DVariant=InternalParameters  IntegratorVariant=Continuous  SatVariant=Disabled  AWVariant=Passthrough  PCopyVariant=Disabled  TRVariant=Disabled  FdbkBlocksVariant=Forward  IdealPFdbkVariant=Disabled  SatFdbkVariant=Disabled  DerivativeFilterVariant=ContFilter  NVariant=InternalParameters  NCopyVariant=Disabled  FilterICVariant=InternalICsFilter  IntegratorICVariant=InternalICs  ExternalResetVariant=Disabled  TRSumVariant=Passthrough  SumFdbkVariant=Disabled  SumVariant=Sum_PID  TsampFilterVariant=InternalTs  TsampNgainVariant=Passthrough  TsampIntegralVariant=Disabled_SignalSpec  ExternalSaturationOutDataTypeStr=Inherit: Same as second input  DerivativeSourceVariant=ErrorSignal  PreIntVariant=InternalPreInt
  PID Controller7 : slpidlib/PID Controller  Commented=on  Controller=PI  Form=Parallel  TimeDomain=Continuous-time  UseExternalTs=off  SampleTime=-1  IntegratorMethod=Forward Euler  FilterMethod=Forward Euler  ControllerParametersSource=internal  P=119.8951  I=54.9494  UseKiTs=off  D=54.9494  UseExternalDerivativeSource=off  N=100  UseFilter=on  TunerSelectOption=Transfer Function Based (PID Tuner App)  InitialConditionSource=internal  InitialConditionForIntegrator=0  InitialConditionForFilter=0  DifferentiatorICPrevScaledInput=0  ExternalReset=none  TrackingMode=off  Kt=1  LimitOutput=off  SatLimitsSource=internal  UpperSaturationLimit=inf  LowerSaturationLimit=-inf  LinearizeAsGain=on  AntiWindupMode=none  Kb=1  LimitIntegrator=off  UpperIntegratorSaturationLimit=inf  LowerIntegratorSaturationLimit=-inf  POutMin=[]  POutMax=[]  IOutMin=[]  IOutMax=[]  DOutMin=[]  DOutMax=[]  NOutMin=[]  NOutMax=[]  SumOutMin=[]  SumOutMax=[]  SaturationOutMin=[]  SaturationOutMax=[]  PParamMin=[]  PParamMax=[]  IParamMin=[]  IParamMax=[]  DParamMin=[]  DParamMax=[]  NParamMin=[]  NParamMax=[]  KbParamMin=[]  KbParamMax=[]  KtParamMin=[]  KtParamMax=[]  KbOutMin=[]  KbOutMax=[]  KtOutMin=[]  KtOutMax=[]  IntegratorOutMin=[]  IntegratorOutMax=[]  FilterOutMin=[]  FilterOutMax=[]  SumI1OutMin=[]  SumI1OutMax=[]  SumI2OutMin=[]  SumI2OutMax=[]  SumI3OutMin=[]  SumI3OutMax=[]  SumI4OutMin=[]  SumI4OutMax=[]  SumDOutMin=[]  SumDOutMax=[]  DifferentiatorOutMin=[]  DifferentiatorOutMax=[]  FilterDiffOutCoefMin=[]  FilterDiffOutCoefMax=[]  ReciprocalOutMin=[]  ReciprocalOutMax=[]  SumDenOutMin=[]  SumDenOutMax=[]  SumNumOutMin=[]  SumNumOutMax=[]  DivideOutMin=[]  DivideOutMax=[]  UdiffTsProdOutMin=[]  UdiffTsProdOutMax=[]  NTsProdOutMin=[]  NTsProdOutMax=[]  UintegralTsProdOutMin=[]  UintegralTsProdOutMax=[]  UngainTsProdOutMin=[]  UngainTsProdOutMax=[]  ClampingZeroOutDataTypeStr=Inherit: Inherit via back propagation  ClampingZeroOutMin=[]  ClampingZeroOutMax=[]  FilterDenConstantOutDataTypeStr=Inherit: Inherit via back propagation  FilterDenConstantOutMin=[]  FilterDenConstantOutMax=[]  PCopyOutDataTypeStr=Inherit: Inherit via back propagation  PCopyOutMin=[]  PCopyOutMax=[]  NCopyOutDataTypeStr=Inherit: Inherit via back propagation  NCopyOutMin=[]  NCopyOutMax=[]  IntegratorContinuousStateAttributes=''  IntegratorStateMustResolveToSignalObject=off  IntegratorRTWStateStorageClass=Auto  FilterContinuousStateAttributes=''  FilterStateMustResolveToSignalObject=off  FilterRTWStateStorageClass=Auto  ParallelPVariant=InternalParameters  IdealPVariant=Disabled  IVariant=InternalParameters  DVariant=Disabled  IntegratorVariant=Continuous  SatVariant=Disabled  AWVariant=Passthrough  PCopyVariant=Disabled  TRVariant=Disabled  FdbkBlocksVariant=Forward  IdealPFdbkVariant=Disabled  SatFdbkVariant=Disabled  DerivativeFilterVariant=Disabled  NVariant=Disabled  NCopyVariant=Disabled_SignalSpec  FilterICVariant=Disabled  IntegratorICVariant=InternalICs  ExternalResetVariant=Disabled  TRSumVariant=Passthrough  SumFdbkVariant=Disabled  SumVariant=Sum_PI  TsampFilterVariant=InternalTs  TsampNgainVariant=Passthrough  TsampIntegralVariant=Disabled_SignalSpec  ExternalSaturationOutDataTypeStr=Inherit: Same as second input  DerivativeSourceVariant=Disabled  PreIntVariant=InternalPreInt
  PID Controller8 : slpidlib/PID Controller  Commented=on  Controller=PI  Form=Parallel  TimeDomain=Continuous-time  UseExternalTs=off  SampleTime=-1  IntegratorMethod=Forward Euler  FilterMethod=Forward Euler  ControllerParametersSource=internal  P=0  I=0.0106816091456831  UseKiTs=off  D=7.9856  UseExternalDerivativeSource=off  N=4.34708219903778  UseFilter=on  TunerSelectOption=Transfer Function Based (PID Tuner App)  InitialConditionSource=internal  InitialConditionForIntegrator=0  InitialConditionForFilter=0  DifferentiatorICPrevScaledInput=0  ExternalReset=none  TrackingMode=off  Kt=1  LimitOutput=off  SatLimitsSource=internal  UpperSaturationLimit=inf  LowerSaturationLimit=-inf  LinearizeAsGain=on  AntiWindupMode=none  Kb=1  LimitIntegrator=off  UpperIntegratorSaturationLimit=inf  LowerIntegratorSaturationLimit=-inf  POutMin=[]  POutMax=[]  IOutMin=[]  IOutMax=[]  DOutMin=[]  DOutMax=[]  NOutMin=[]  NOutMax=[]  SumOutMin=[]  SumOutMax=[]  SaturationOutMin=[]  SaturationOutMax=[]  PParamMin=[]  PParamMax=[]  IParamMin=[]  IParamMax=[]  DParamMin=[]  DParamMax=[]  NParamMin=[]  NParamMax=[]  KbParamMin=[]  KbParamMax=[]  KtParamMin=[]  KtParamMax=[]  KbOutMin=[]  KbOutMax=[]  KtOutMin=[]  KtOutMax=[]  IntegratorOutMin=[]  IntegratorOutMax=[]  FilterOutMin=[]  FilterOutMax=[]  SumI1OutMin=[]  SumI1OutMax=[]  SumI2OutMin=[]  SumI2OutMax=[]  SumI3OutMin=[]  SumI3OutMax=[]  SumI4OutMin=[]  SumI4OutMax=[]  SumDOutMin=[]  SumDOutMax=[]  DifferentiatorOutMin=[]  DifferentiatorOutMax=[]  FilterDiffOutCoefMin=[]  FilterDiffOutCoefMax=[]  ReciprocalOutMin=[]  ReciprocalOutMax=[]  SumDenOutMin=[]  SumDenOutMax=[]  SumNumOutMin=[]  SumNumOutMax=[]  DivideOutMin=[]  DivideOutMax=[]  UdiffTsProdOutMin=[]  UdiffTsProdOutMax=[]  NTsProdOutMin=[]  NTsProdOutMax=[]  UintegralTsProdOutMin=[]  UintegralTsProdOutMax=[]  UngainTsProdOutMin=[]  UngainTsProdOutMax=[]  ClampingZeroOutDataTypeStr=Inherit: Inherit via back propagation  ClampingZeroOutMin=[]  ClampingZeroOutMax=[]  FilterDenConstantOutDataTypeStr=Inherit: Inherit via back propagation  FilterDenConstantOutMin=[]  FilterDenConstantOutMax=[]  PCopyOutDataTypeStr=Inherit: Inherit via back propagation  PCopyOutMin=[]  PCopyOutMax=[]  NCopyOutDataTypeStr=Inherit: Inherit via back propagation  NCopyOutMin=[]  NCopyOutMax=[]  IntegratorContinuousStateAttributes=''  IntegratorStateMustResolveToSignalObject=off  IntegratorRTWStateStorageClass=Auto  FilterContinuousStateAttributes=''  FilterStateMustResolveToSignalObject=off  FilterRTWStateStorageClass=Auto  ParallelPVariant=InternalParameters  IdealPVariant=Disabled  IVariant=InternalParameters  DVariant=Disabled  IntegratorVariant=Continuous  SatVariant=Disabled  AWVariant=Passthrough  PCopyVariant=Disabled  TRVariant=Disabled  FdbkBlocksVariant=Forward  IdealPFdbkVariant=Disabled  SatFdbkVariant=Disabled  DerivativeFilterVariant=Disabled  NVariant=Disabled  NCopyVariant=Disabled_SignalSpec  FilterICVariant=Disabled  IntegratorICVariant=InternalICs  ExternalResetVariant=Disabled  TRSumVariant=Passthrough  SumFdbkVariant=Disabled  SumVariant=Sum_PI  TsampFilterVariant=InternalTs  TsampNgainVariant=Passthrough  TsampIntegralVariant=Disabled_SignalSpec  ExternalSaturationOutDataTypeStr=Inherit: Same as second input  DerivativeSourceVariant=Disabled  PreIntVariant=InternalPreInt
  PID Controller9 : slpidlib/PID Controller  Commented=on  Controller=PD  Form=Parallel  TimeDomain=Continuous-time  UseExternalTs=off  SampleTime=-1  IntegratorMethod=Forward Euler  FilterMethod=Forward Euler  ControllerParametersSource=internal  P=0.527513707722222  I=1  UseKiTs=off  D=0.744390768544689  UseExternalDerivativeSource=off  N=11.0148881441152  UseFilter=on  TunerSelectOption=Transfer Function Based (PID Tuner App)  InitialConditionSource=internal  InitialConditionForIntegrator=0  InitialConditionForFilter=0  DifferentiatorICPrevScaledInput=0  ExternalReset=none  TrackingMode=off  Kt=1  LimitOutput=off  SatLimitsSource=internal  UpperSaturationLimit=inf  LowerSaturationLimit=-inf  LinearizeAsGain=on  AntiWindupMode=none  Kb=1  LimitIntegrator=off  UpperIntegratorSaturationLimit=inf  LowerIntegratorSaturationLimit=-inf  POutMin=[]  POutMax=[]  IOutMin=[]  IOutMax=[]  DOutMin=[]  DOutMax=[]  NOutMin=[]  NOutMax=[]  SumOutMin=[]  SumOutMax=[]  SaturationOutMin=[]  SaturationOutMax=[]  PParamMin=[]  PParamMax=[]  IParamMin=[]  IParamMax=[]  DParamMin=[]  DParamMax=[]  NParamMin=[]  NParamMax=[]  KbParamMin=[]  KbParamMax=[]  KtParamMin=[]  KtParamMax=[]  KbOutMin=[]  KbOutMax=[]  KtOutMin=[]  KtOutMax=[]  IntegratorOutMin=[]  IntegratorOutMax=[]  FilterOutMin=[]  FilterOutMax=[]  SumI1OutMin=[]  SumI1OutMax=[]  SumI2OutMin=[]  SumI2OutMax=[]  SumI3OutMin=[]  SumI3OutMax=[]  SumI4OutMin=[]  SumI4OutMax=[]  SumDOutMin=[]  SumDOutMax=[]  DifferentiatorOutMin=[]  DifferentiatorOutMax=[]  FilterDiffOutCoefMin=[]  FilterDiffOutCoefMax=[]  ReciprocalOutMin=[]  ReciprocalOutMax=[]  SumDenOutMin=[]  SumDenOutMax=[]  SumNumOutMin=[]  SumNumOutMax=[]  DivideOutMin=[]  DivideOutMax=[]  UdiffTsProdOutMin=[]  UdiffTsProdOutMax=[]  NTsProdOutMin=[]  NTsProdOutMax=[]  UintegralTsProdOutMin=[]  UintegralTsProdOutMax=[]  UngainTsProdOutMin=[]  UngainTsProdOutMax=[]  ClampingZeroOutDataTypeStr=Inherit: Inherit via back propagation  ClampingZeroOutMin=[]  ClampingZeroOutMax=[]  FilterDenConstantOutDataTypeStr=Inherit: Inherit via back propagation  FilterDenConstantOutMin=[]  FilterDenConstantOutMax=[]  PCopyOutDataTypeStr=Inherit: Inherit via back propagation  PCopyOutMin=[]  PCopyOutMax=[]  NCopyOutDataTypeStr=Inherit: Inherit via back propagation  NCopyOutMin=[]  NCopyOutMax=[]  IntegratorContinuousStateAttributes=''  IntegratorStateMustResolveToSignalObject=off  IntegratorRTWStateStorageClass=Auto  FilterContinuousStateAttributes=''  FilterStateMustResolveToSignalObject=off  FilterRTWStateStorageClass=Auto  ParallelPVariant=InternalParameters  IdealPVariant=Disabled  IVariant=Disabled  DVariant=InternalParameters  IntegratorVariant=Disabled  SatVariant=Disabled  AWVariant=Disabled  PCopyVariant=Disabled  TRVariant=Disabled  FdbkBlocksVariant=Forward  IdealPFdbkVariant=Disabled  SatFdbkVariant=Disabled  DerivativeFilterVariant=ContFilter  NVariant=InternalParameters  NCopyVariant=Disabled  FilterICVariant=InternalICsFilter  IntegratorICVariant=Disabled  ExternalResetVariant=Disabled  TRSumVariant=Passthrough  SumFdbkVariant=Disabled  SumVariant=Sum_PD  TsampFilterVariant=InternalTs  TsampNgainVariant=Passthrough  TsampIntegralVariant=Disabled_SignalSpec  ExternalSaturationOutDataTypeStr=Inherit: Same as second input  DerivativeSourceVariant=ErrorSignal  PreIntVariant=InternalPreInt
  Pitch : Scope
  Pitch1 : Scope  Commented=on
  Position wrt earth1 : MATLAB Function  Commented=on  TreatAsAtomicUnit=on
  Position wrt earth2 : MATLAB Function  Commented=on  TreatAsAtomicUnit=on
  Position wrt earth3 : MATLAB Function  Commented=on  TreatAsAtomicUnit=on
  Position wrt earth4 : MATLAB Function  Commented=on  TreatAsAtomicUnit=on
  Radians to Degrees : simulink_extras/Transformations/Radians to Degrees
  Radians to Degrees1 : simulink_extras/Transformations/Radians to Degrees
  Radians to Degrees2 : simulink_extras/Transformations/Radians to Degrees  Commented=on
  Radians to Degrees3 : simulink_extras/Transformations/Radians to Degrees  Commented=on
  Scope{,1..5,7..8,18} (9 alike) : Scope  Commented=on  NumInputPorts=3
  Scope10 : Scope
  Scope{6,9,11..17,19..20} (11 alike) : Scope  Commented=on
  Simulation 3D Camera : sim3dcameralib/Simulation 3D Camera  Priority=1  Commented=on  sensorTag=Sim3dSensor�  sensorId=1  sensorName=Sim3dSensor�  vehTagList={'Scene Origin';'SimulinkVehicle1'}  vehTag=SimulinkVehicle1  mountLoc=Origin  offsetFlag=on  tmountOffset=[0, 0, 0]  extTmount=off  rmountOffset=[0, 0, 0]  extRmount=off  FocalLength=[1109, 1109]  OpticalCenter=[640, 360]  ImageSize=[720, 1280]  RadialDistortion=[0, 0]  TangentialDistortion=[0, 0]  SensorSkew=0  DepthOutportEnabled=off  SemanticOutportEnabled=off  TransformOutportEnabled=off  SampleTime=-1  mountPoint=[0 0 0]  mountOrientation=[0 0 0]  aMode=4  ID=1
      settings: LibrarySourceBlock=uavsim3dlib/Simulation 3D Camera
  Simulation 3D Scene Configuration : sim3dlib/Simulation 3D Scene Configuration  Priority=0  Commented=on  ProjectFormat=Default Scenes  SceneDesc=US city block  ProjectName=C:\Program Files\MATLAB\R2024b\toolbox\shared\sim3d_projects\automotive_project_windows\UE\WindowsNoEditor\VehicleSimulation.exe  ScenePath=/Game/Maps/USCityBlock  EnableOpenDRIVE=off  vehTagList={'Custom';'Scene Origin';'SimulinkVehicle1'}  vehTag=SimulinkVehicle1  FreeCameraInitialTranslation=[0, 0, 0]  FreeCameraDefaultInitialTranslation=[-6, 0, 2]  FreeCameraInitialRotation=[0, 0, 0]  FreeCameraDefaultInitialRotation=[0, -15, 0]  OpVisEn=off  Ts=0.1  EnableWindow=on  EnableRemoteAccess=off  EnableWeather=off  SunAzimuth=90  SunAltitude=40.0  EnableGeospatialSun=off  Latitude=0  Longitude=0  Date=2023-01-01  Time=10:30:00  GeoTimeZone=-5.0  SunDaylightSaving=off  wind=1  clouds=10  EnableVolumetricClouds=off  CloudCoverage=0  CloudAltitude=6  fog=0  rain=0  RaindropsEffect=off  SnowDensity=0  EnableGeospatial=off  UseTrueOrigin=off  OriginHeight=200  OriginLatitude=40.744652  OriginLongitude=-73.988864  MapStyle=Aerial  AdditionalAssetIDs=[]  UseAdvancedSunSky=off  SolarTime=11  TimeZone=-5  Day=21  Month=9  Year=2022  UseDaylightSavingTime=on  DSTStartDay=10  DSTStartMonth=3  DSTEndDay=3  DSTEndMonth=11  DSTSwitchHour=2  sensorTag=MainCamera1  sensorId=1  sensorName=MainCamera1  mountLoc=Origin  offsetFlag=off  tmountOffset=[0, 0, 0]  rmountOffset=[0, 0, 0]  HorizontalResolution=1280  VerticalResolution=720  HorizontalFOV=60  mountPoint=[0 0 0]  mountOrientation=[0 0 0]  aMode=4  ID=1  GeoTrigger=Inactive
      settings: LibrarySourceBlock=uavsim3dlib/Simulation 3D Scene Configuration
  Simulation 3D UAV Vehicle : uavsim3dlib/Simulation 3D UAV Vehicle  Priority=-1  Commented=on  Mesh=Custom  MeshPath=C:\Users\nicol\OneDrive - Stellenbosch University\uni\Meesters\Blender\untitled.fbx  Color=Black  ActorName=SimulinkVehicle1  UseGlobalFrame=on  InitialTranslation=[0 0 0]  InitialRotation=[0 0 0]  InitialTranslationGlobal=[0 0 0]  InitialGeoOrigin=[0 0 0]  InitialRotationGlobal=[0 0 0]  SampleTime=-1  ActorType=SimulinkVehicle  ID=1  aMode=4  ActorTag=SimulinkVehicle1
  Step : Step  Commented=on  SampleTime=0
  Step1 : Step  Commented=on  Time=0  After=0  SampleTime=0
  Step2 : Step  After=-5  SampleTime=0
  Step3 : Step  Commented=on  SampleTime=0
  Step4 : Step  Time=20  After=5  SampleTime=0
  Sum{,1,3..10,12} (11 alike) : Sum  Commented=on  Inputs=|+-
  Sum11 : Sum  Inputs=|++
  Sum2 : Sum  Inputs=|+-
  To Workspace : ToWorkspace  Commented=on  VariableName=XYZ  SaveFormat=Timeseries  SampleTime=t_s
  To Workspace1 : ToWorkspace  VariableName=u  SaveFormat=Timeseries  SampleTime=0.01
  To Workspace2 : ToWorkspace  VariableName=pitch  SaveFormat=Timeseries  SampleTime=-1
  To Workspace3 : ToWorkspace  Commented=on  VariableName=u1  SaveFormat=Timeseries  SampleTime=0.01
  To Workspace4 : ToWorkspace  VariableName=delta_e_ref  SaveFormat=Timeseries  SampleTime=0.001
  To Workspace5 : ToWorkspace  VariableName=Z  SaveFormat=Timeseries  SampleTime=0.001
  To Workspace6 : ToWorkspace  Commented=on  VariableName=EA  SaveFormat=Timeseries  SampleTime=t_s
  Transfer Fcn : TransferFcn  Commented=on  Numerator=[-2.053e-05 0.01595]  Denominator=[1 0.356 0.0007681]
  Transfer Fcn2 : TransferFcn  Commented=on  Numerator=[-2.053e-05 0.01595]  Denominator=[1 0.356 0.0007681]
  Vel_FNL : slpidlib/PID Controller  Commented=on  Controller=PI  Form=Parallel  TimeDomain=Continuous-time  UseExternalTs=off  SampleTime=-1  IntegratorMethod=Forward Euler  FilterMethod=Forward Euler  ControllerParametersSource=internal  P=119.8951  I=54.9494  UseKiTs=off  D=54.9494  UseExternalDerivativeSource=off  N=100  UseFilter=on  TunerSelectOption=Transfer Function Based (PID Tuner App)  InitialConditionSource=internal  InitialConditionForIntegrator=0  InitialConditionForFilter=0  DifferentiatorICPrevScaledInput=0  ExternalReset=none  TrackingMode=off  Kt=1  LimitOutput=off  SatLimitsSource=internal  UpperSaturationLimit=inf  LowerSaturationLimit=-inf  LinearizeAsGain=on  AntiWindupMode=none  Kb=1  LimitIntegrator=off  UpperIntegratorSaturationLimit=inf  LowerIntegratorSaturationLimit=-inf  POutMin=[]  POutMax=[]  IOutMin=[]  IOutMax=[]  DOutMin=[]  DOutMax=[]  NOutMin=[]  NOutMax=[]  SumOutMin=[]  SumOutMax=[]  SaturationOutMin=[]  SaturationOutMax=[]  PParamMin=[]  PParamMax=[]  IParamMin=[]  IParamMax=[]  DParamMin=[]  DParamMax=[]  NParamMin=[]  NParamMax=[]  KbParamMin=[]  KbParamMax=[]  KtParamMin=[]  KtParamMax=[]  KbOutMin=[]  KbOutMax=[]  KtOutMin=[]  KtOutMax=[]  IntegratorOutMin=[]  IntegratorOutMax=[]  FilterOutMin=[]  FilterOutMax=[]  SumI1OutMin=[]  SumI1OutMax=[]  SumI2OutMin=[]  SumI2OutMax=[]  SumI3OutMin=[]  SumI3OutMax=[]  SumI4OutMin=[]  SumI4OutMax=[]  SumDOutMin=[]  SumDOutMax=[]  DifferentiatorOutMin=[]  DifferentiatorOutMax=[]  FilterDiffOutCoefMin=[]  FilterDiffOutCoefMax=[]  ReciprocalOutMin=[]  ReciprocalOutMax=[]  SumDenOutMin=[]  SumDenOutMax=[]  SumNumOutMin=[]  SumNumOutMax=[]  DivideOutMin=[]  DivideOutMax=[]  UdiffTsProdOutMin=[]  UdiffTsProdOutMax=[]  NTsProdOutMin=[]  NTsProdOutMax=[]  UintegralTsProdOutMin=[]  UintegralTsProdOutMax=[]  UngainTsProdOutMin=[]  UngainTsProdOutMax=[]  ClampingZeroOutDataTypeStr=Inherit: Inherit via back propagation  ClampingZeroOutMin=[]  ClampingZeroOutMax=[]  FilterDenConstantOutDataTypeStr=Inherit: Inherit via back propagation  FilterDenConstantOutMin=[]  FilterDenConstantOutMax=[]  PCopyOutDataTypeStr=Inherit: Inherit via back propagation  PCopyOutMin=[]  PCopyOutMax=[]  NCopyOutDataTypeStr=Inherit: Inherit via back propagation  NCopyOutMin=[]  NCopyOutMax=[]  IntegratorContinuousStateAttributes=''  IntegratorStateMustResolveToSignalObject=off  IntegratorRTWStateStorageClass=Auto  FilterContinuousStateAttributes=''  FilterStateMustResolveToSignalObject=off  FilterRTWStateStorageClass=Auto  ParallelPVariant=InternalParameters  IdealPVariant=Disabled  IVariant=InternalParameters  DVariant=Disabled  IntegratorVariant=Continuous  SatVariant=Disabled  AWVariant=Passthrough  PCopyVariant=Disabled  TRVariant=Disabled  FdbkBlocksVariant=Forward  IdealPFdbkVariant=Disabled  SatFdbkVariant=Disabled  DerivativeFilterVariant=Disabled  NVariant=Disabled  NCopyVariant=Disabled_SignalSpec  FilterICVariant=Disabled  IntegratorICVariant=InternalICs  ExternalResetVariant=Disabled  TRSumVariant=Passthrough  SumFdbkVariant=Disabled  SumVariant=Sum_PI  TsampFilterVariant=InternalTs  TsampNgainVariant=Passthrough  TsampIntegralVariant=Disabled_SignalSpec  ExternalSaturationOutDataTypeStr=Inherit: Same as second input  DerivativeSourceVariant=Disabled  PreIntVariant=InternalPreInt
  "Velocity transfer function " : TransferFcn  Commented=on  Numerator=[0.13345]  Denominator=[1 0.667]
  Video Viewer : VideoViewer  Commented=on  FigPos=[955 1030 958 925]
  X Y Z : Scope  Commented=on
  XYZ : Scope  NumInputPorts=3
  XYZ1 : Scope  Commented=on  NumInputPorts=3
  YAW : Constant  Commented=on  Value=10
  nonlinear dynamics piecewise : Subsystem  Commented=on
  nonlinear dynamics piecewise1 : Subsystem  Commented=on
  nonlinear dynamics piecewise2 : Subsystem  Commented=on
  position rate wrt Earth : MATLABFcn  Commented=on  MATLABFcn=position_wrt_Earth  OutputDimensions=3
  uvw : Scope  NumInputPorts=3
  uvw1 : Scope  Commented=on  NumInputPorts=3
  yaw : Scope
  yaw1 : Scope  Commented=on
  yaw_FNL : slpidlib/PID Controller  Commented=on  Controller=PD  Form=Parallel  TimeDomain=Continuous-time  UseExternalTs=off  SampleTime=-1  IntegratorMethod=Forward Euler  FilterMethod=Forward Euler  ControllerParametersSource=internal  P=0.115369751085597  I=0  UseKiTs=off  D=0.178743752919418  UseExternalDerivativeSource=off  N=1.68043173640321  UseFilter=on  TunerSelectOption=Transfer Function Based (PID Tuner App)  InitialConditionSource=internal  InitialConditionForIntegrator=0  InitialConditionForFilter=0  DifferentiatorICPrevScaledInput=0  ExternalReset=none  TrackingMode=off  Kt=1  LimitOutput=off  SatLimitsSource=internal  UpperSaturationLimit=inf  LowerSaturationLimit=-inf  LinearizeAsGain=on  AntiWindupMode=none  Kb=1  LimitIntegrator=off  UpperIntegratorSaturationLimit=inf  LowerIntegratorSaturationLimit=-inf  POutMin=[]  POutMax=[]  IOutMin=[]  IOutMax=[]  DOutMin=[]  DOutMax=[]  NOutMin=[]  NOutMax=[]  SumOutMin=[]  SumOutMax=[]  SaturationOutMin=[]  SaturationOutMax=[]  PParamMin=[]  PParamMax=[]  IParamMin=[]  IParamMax=[]  DParamMin=[]  DParamMax=[]  NParamMin=[]  NParamMax=[]  KbParamMin=[]  KbParamMax=[]  KtParamMin=[]  KtParamMax=[]  KbOutMin=[]  KbOutMax=[]  KtOutMin=[]  KtOutMax=[]  IntegratorOutMin=[]  IntegratorOutMax=[]  FilterOutMin=[]  FilterOutMax=[]  SumI1OutMin=[]  SumI1OutMax=[]  SumI2OutMin=[]  SumI2OutMax=[]  SumI3OutMin=[]  SumI3OutMax=[]  SumI4OutMin=[]  SumI4OutMax=[]  SumDOutMin=[]  SumDOutMax=[]  DifferentiatorOutMin=[]  DifferentiatorOutMax=[]  FilterDiffOutCoefMin=[]  FilterDiffOutCoefMax=[]  ReciprocalOutMin=[]  ReciprocalOutMax=[]  SumDenOutMin=[]  SumDenOutMax=[]  SumNumOutMin=[]  SumNumOutMax=[]  DivideOutMin=[]  DivideOutMax=[]  UdiffTsProdOutMin=[]  UdiffTsProdOutMax=[]  NTsProdOutMin=[]  NTsProdOutMax=[]  UintegralTsProdOutMin=[]  UintegralTsProdOutMax=[]  UngainTsProdOutMin=[]  UngainTsProdOutMax=[]  ClampingZeroOutDataTypeStr=Inherit: Inherit via back propagation  ClampingZeroOutMin=[]  ClampingZeroOutMax=[]  FilterDenConstantOutDataTypeStr=Inherit: Inherit via back propagation  FilterDenConstantOutMin=[]  FilterDenConstantOutMax=[]  PCopyOutDataTypeStr=Inherit: Inherit via back propagation  PCopyOutMin=[]  PCopyOutMax=[]  NCopyOutDataTypeStr=Inherit: Inherit via back propagation  NCopyOutMin=[]  NCopyOutMax=[]  IntegratorContinuousStateAttributes=''  IntegratorStateMustResolveToSignalObject=off  IntegratorRTWStateStorageClass=Auto  FilterContinuousStateAttributes=''  FilterStateMustResolveToSignalObject=off  FilterRTWStateStorageClass=Auto  ParallelPVariant=InternalParameters  IdealPVariant=Disabled  IVariant=Disabled  DVariant=InternalParameters  IntegratorVariant=Disabled  SatVariant=Disabled  AWVariant=Disabled  PCopyVariant=Disabled  TRVariant=Disabled  FdbkBlocksVariant=Forward  IdealPFdbkVariant=Disabled  SatFdbkVariant=Disabled  DerivativeFilterVariant=ContFilter  NVariant=InternalParameters  NCopyVariant=Disabled  FilterICVariant=InternalICsFilter  IntegratorICVariant=Disabled  ExternalResetVariant=Disabled  TRSumVariant=Passthrough  SumFdbkVariant=Disabled  SumVariant=Sum_PD  TsampFilterVariant=InternalTs  TsampNgainVariant=Passthrough  TsampIntegralVariant=Disabled_SignalSpec  ExternalSaturationOutDataTypeStr=Inherit: Same as second input  DerivativeSourceVariant=ErrorSignal  PreIntVariant=InternalPreInt
  wires:
  Euler angle rate/1 -> Integrator1/1
  Integrator1/1 -> Euler angles/1, Mux/1, Mux2/2, Mux1/2  "Phi, theta, psi"
  Integrator/1 -> Mux2/1, Mux1/1, Mux/2  "u, v, w, p ,q, r"
  Mux/1 -> Euler angle rate/1  "phi theta psi u v w p q r"
  Mux1/1 -> position rate wrt Earth/1
  position rate wrt Earth/1 -> Integrator2/1
  Integrator2/1 -> X Y Z/1, Mux2/3  "X, Y, Z"
  Mux2/1 -> "Dynamic equation of motion u_dot, v_dot, w_dot, p_dot, q_dot, r_dot"/1
  "Dynamic equation of motion u_dot, v_dot, w_dot, p_dot, q_dot, r_dot"/1 -> Integrator/1
  Demux5/2 -> Scope1/2, Nonlinear dynamics1/11(YE)
  Demux5/3 -> Scope1/3, Nonlinear dynamics1/12(ZE)
  Demux4/3 -> Scope/3, Nonlinear dynamics1/9(psi), Euler angle estimation1/3(psi), Position wrt earth1/6(psi)
  Integrator6/1 -> Demux3/1
  Demux3/1 -> Nonlinear dynamics1/1(u), Position wrt earth1/1(u)
  Integrator7/1 -> Demux4/1
  Demux3/6 -> Nonlinear dynamics1/6(r), Euler angle estimation1/6(r)
  Demux3/4 -> Nonlinear dynamics1/4(p), Euler angle estimation1/4(p)
  Euler angle estimation1/1(EA_dot) -> Integrator7/1
  Demux5/1 -> Scope1/1, Nonlinear dynamics1/10(XE)
  Demux4/1 -> Scope/1, Nonlinear dynamics1/7(phi), Position wrt earth1/4(phi), Euler angle estimation1/1(phi)
  Demux3/5 -> Nonlinear dynamics1/5(q), Euler angle estimation1/5(q)
  Demux3/2 -> Nonlinear dynamics1/2(v), Position wrt earth1/2(v)
  Position wrt earth1/1(XYZ_dot) -> Integrator8/1
  Demux4/2 -> Scope/2, Nonlinear dynamics1/8(theta), Euler angle estimation1/2(theta), Position wrt earth1/5(theta)
  Demux3/3 -> Nonlinear dynamics1/3(w), Position wrt earth1/3(w)
  Integrator8/1 -> Demux5/1
  Nonlinear dynamics1/1(V_dot) -> Integrator6/1
  Constant/1 -> Nonlinear dynamics1/13(MAF)
  nonlinear dynamics piecewise/1(V_dot) -> Integrator3/1
  Demux1/5 -> nonlinear dynamics piecewise/5(In5), Euler angle estimation2/5(q)
  Integrator3/1 -> Demux1/1
  Demux2/1 -> Scope2/1, nonlinear dynamics piecewise/7(In7), Position wrt earth2/4(phi), Euler angle estimation2/1(phi)
  Demux6/2 -> nonlinear dynamics piecewise/11(In11), Scope3/2
  Demux1/3 -> nonlinear dynamics piecewise/3(In3), Position wrt earth2/3(w)
  Demux1/4 -> nonlinear dynamics piecewise/4(In4), Euler angle estimation2/4(p)
  Position wrt earth2/1(XYZ_dot) -> Integrator5/1
  Demux2/3 -> Scope2/3, nonlinear dynamics piecewise/9(In9), Euler angle estimation2/3(psi), Position wrt earth2/6(psi)
  Demux6/3 -> nonlinear dynamics piecewise/12(In12), Scope3/3
  Integrator5/1 -> Demux6/1
  Demux1/1 -> nonlinear dynamics piecewise/1(In1), Position wrt earth2/1(u)
  Demux6/1 -> nonlinear dynamics piecewise/10(In10), Scope3/1
  Integrator4/1 -> Demux2/1
  Demux1/2 -> nonlinear dynamics piecewise/2(In2), Position wrt earth2/2(v)
  Euler angle estimation2/1(EA_dot) -> Integrator4/1
  Demux2/2 -> Scope2/2, nonlinear dynamics piecewise/8(In8), Position wrt earth2/5(theta), Euler angle estimation2/2(theta)
  Demux1/6 -> nonlinear dynamics piecewise/6(In6), Euler angle estimation2/6(r)
  Demux8/1 -> Scope4/1, nonlinear dynamics piecewise1/7(In7), Position wrt earth3/4(phi), Euler angle estimation3/1(phi)
  Demux7/1 -> Integrator9/1
  Integrator10/1 -> To Workspace6/1, Simulation 3D UAV Vehicle/2, Demux8/1
  Demux7/2 -> Integrator12/1
  Demux9/3 -> nonlinear dynamics piecewise1/12(In12), Multiply/1
  Demux7/4 -> Integrator14/1
  Euler angle estimation3/1(EA_dot) -> Integrator10/1
  Demux9/1 -> Mux3/1, Scope5/1, nonlinear dynamics piecewise1/10(In10)
  Demux7/6 -> Integrator16/1
  Integrator11/1 -> To Workspace/1, Demux9/1
  nonlinear dynamics piecewise1/1(V_dot) -> Demux7/1
  Demux7/3 -> Integrator13/1
  Demux9/2 -> nonlinear dynamics piecewise1/11(In11), Mux3/2, Scope5/2
  Demux8/2 -> Scope4/2, nonlinear dynamics piecewise1/8(In8), Position wrt earth3/5(theta), Euler angle estimation3/2(theta)
  Position wrt earth3/1(XYZ_dot) -> Integrator11/1
  Demux7/5 -> Integrator15/1
  Demux8/3 -> Scope4/3, nonlinear dynamics piecewise1/9(In9), Euler angle estimation3/3(psi), Position wrt earth3/6(psi)
  Integrator9/1 -> nonlinear dynamics piecewise1/1(In1), Scope6/1, Position wrt earth3/1(u), Scope18/1
  Integrator12/1 -> nonlinear dynamics piecewise1/2(In2), Scope18/2, Position wrt earth3/2(v)
  Integrator14/1 -> Euler angle estimation3/4(p), nonlinear dynamics piecewise1/4(In4)
  Integrator13/1 -> nonlinear dynamics piecewise1/3(In3), Scope18/3, Position wrt earth3/3(w)
  Integrator15/1 -> Euler angle estimation3/5(q), nonlinear dynamics piecewise1/5(In5)
  Integrator16/1 -> Euler angle estimation3/6(r), nonlinear dynamics piecewise1/6(In6)
  Demux11/3 -> Scope7/3, Euler angle estimation4/3(psi), Position wrt earth4/6(psi), nonlinear dynamics piecewise2/9(In9)
  Position wrt earth4/1(XYZ_dot) -> Integrator18/1
  Integrator24/1 -> nonlinear dynamics piecewise2/1(u), Scope9/1, Position wrt earth4/1(u)
  Demux10/6 -> Integrator23/1
  Demux10/1 -> Integrator24/1
  Demux12/1 -> Scope8/1
  Demux11/1 -> Scope7/1, nonlinear dynamics piecewise2/7(phi), Position wrt earth4/4(phi), Euler angle estimation4/1(phi)
  Integrator23/1 -> Euler angle estimation4/6(r), nonlinear dynamics piecewise2/6(r)
  Demux10/2 -> Integrator19/1
  nonlinear dynamics piecewise2/1(V_dot) -> Demux10/1
  Demux12/3 -> nonlinear dynamics piecewise2/10(Z), Scope8/3
  Integrator20/1 -> nonlinear dynamics piecewise2/3(w), Position wrt earth4/3(w)
  Integrator21/1 -> Euler angle estimation4/4(p), nonlinear dynamics piecewise2/4(p)
  Euler angle estimation4/1(EA_dot) -> Integrator17/1
  Demux10/4 -> Integrator21/1
  Integrator17/1 -> Demux11/1
  Demux10/3 -> Integrator20/1
  Integrator22/1 -> Euler angle estimation4/5(q), nonlinear dynamics piecewise2/5(q)
  Demux12/2 -> Scope8/2
  Demux10/5 -> Integrator22/1
  Integrator19/1 -> nonlinear dynamics piecewise2/2(v), Position wrt earth4/2(v)
  Demux11/2 -> Scope7/2, nonlinear dynamics piecewise2/8(theta), Position wrt earth4/5(theta), Euler angle estimation4/2(theta)
  Integrator18/1 -> Demux12/1
  Simulation 3D Camera/1 -> Video Viewer/1
  Multiply/1 -> Scope5/3, Mux3/3
  Mux3/1 -> Simulation 3D UAV Vehicle/1
  Constant7/1 -> Airship_model/3(prop1_alpha)
  Constant8/1 -> Airship_model/4(prop2_alpha)
  Airship_model/1(EA) -> EA/1, Demux/1
  Demux/3 -> Radians to Degrees/1
  Demux13/1 -> XYZ/1
  Demux13/2 -> XYZ/2
  Demux13/3 -> Gain/1
  Airship_model/2(XYZ) -> Demux13/1
  Demux/2 -> Radians to Degrees1/1
  Radians to Degrees1/1 -> To Workspace2/1, Pitch/1
  Sum2/1 -> PID Controller3/1, PID Controller2/1
  Constant5/1 -> Sum2/1
  Airship_model/3(uvw) -> Demux14/1
  Demux14/1 -> To Workspace1/1, Sum2/2, uvw/1
  Demux14/2 -> uvw/2
  Demux14/3 -> uvw/3
  Airship_model1/2(XYZ) -> Demux16/1
  Demux17/1 -> Sum5/2, To Workspace3/1, uvw1/1
  Constant6/1 -> Airship_model1/4(prop2_alpha)
  Step1/1 -> Scope14/1, Sum4/1
  Airship_model1/1(EA) -> EA1/1, Demux15/1
  Sum3/1 -> yaw_FNL/1
  Demux16/2 -> XYZ1/2
  Sum4/1 -> PID Controller5/1
  Gain2/1 -> XYZ1/3
  Radians to Degrees3/1 -> Sum4/2, Pitch1/1
  Constant4/1 -> Airship_model1/3(prop1_alpha)
  Demux16/1 -> XYZ1/1
  Demux16/3 -> Gain2/1
  Demux15/3 -> Radians to Degrees2/1
  Demux17/2 -> uvw1/2
  Demux17/3 -> uvw1/3
  Demux15/2 -> Radians to Degrees3/1
  PID Controller5/1 -> Airship_model1/5(delta_e)
  Airship_model1/3(uvw) -> Demux17/1
  Constant1/1 -> Sum3/1
  Radians to Degrees2/1 -> Sum3/2, yaw1/1
  Vel_FNL/1 -> Airship_model1/1(fProp1), Airship_model1/2(fProp2)
  Sum5/1 -> Vel_FNL/1
  Constant2/1 -> Sum5/1
  Constant9/1 -> Sum6/1
  Sum6/1 -> PID Controller7/1
  "Velocity transfer function "/1 -> Sum6/2, Scope15/1
  PID Controller7/1 -> "Velocity transfer function "/1
  Constant10/1 -> Airship_model/1(fProp1)
  Constant11/1 -> Airship_model/2(fProp2)
  yaw_FNL/1 -> Airship_model1/6(delta_r)
  Sum/1 -> PID Controller/1
  YAW/1 -> Sum/1
  PID Controller/1 -> 10deg 2 zeros/1
  10deg 2 zeros/1 -> Sum/2, Scope12/1
  10deg 3 zeros/1 -> Sum1/2, Scope13/1
  PID Controller1/1 -> 10deg 3 zeros/1
  Constant12/1 -> Sum1/1
  Sum1/1 -> PID Controller1/1
  Clock1/1 -> MATLAB Function/1(t)
  Constant13/1 -> Sum7/1
  Sum7/1 -> PID Controller8/1
  PID Controller8/1 -> Chirp TF/1
  Chirp TF/1 -> Sum7/2, Scope16/1
  PID Controller9/1 -> 5deg 2 zeros/1
  5deg 2 zeros/1 -> Sum8/2, Scope17/1
  Sum8/1 -> PID Controller9/1
  Constant14/1 -> Sum8/1
  PID Controller10/1 -> "2 and 5deg mix "/1
  "2 and 5deg mix "/1 -> Sum9/2, Scope11/1
  Sum9/1 -> PID Controller10/1
  Constant15/1 -> Sum9/1
  Radians to Degrees/1 -> yaw/1
  Constant3/1 -> Airship_model/6(delta_r)
  PID Controller4/1 -> Transfer Fcn/1
  Sum10/1 -> PID Controller4/1
  Transfer Fcn/1 -> Sum10/2, Scope19/1
  Step/1 -> Sum10/1
  Gain/1 -> To Workspace5/1, Altitude/1, XYZ/3
  MATLAB Function/1(y) -> Scope10/1, To Workspace4/1
  Sum12/1 -> PID Controller11/1
  Step3/1 -> Sum12/1
  Transfer Fcn2/1 -> Sum12/2, Scope20/1
  PID Controller11/1 -> Transfer Fcn2/1
  Step2/1 -> Sum11/1
  Step4/1 -> Sum11/2
  Sum11/1 -> Airship_model/5(delta_e)
